simulink model "chap2_2"  (Simulink 3.00)
settings: Solver=ode4  StartTime=0  StopTime=2  FixedStep=0.001  RelTol=1e-3
settings Model: SaveTime=off  SaveOutput=off  LastModifiedBy=liu

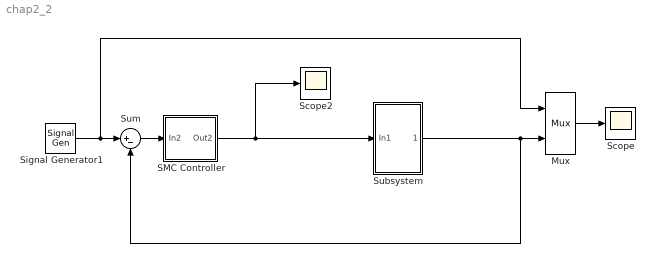
== system chap2_2 ==
  Mux : Mux  Inputs=2
      settings: DisplayOption=none
  SMC Controller : Subsystem
  Scope : Scope
      settings: TimeRange=1  YMin=-0.55  YMax=0.55  SaveName=datas  MaxRows=500000
  Scope2 : Scope
      settings: TimeRange=auto  YMin=-5  YMax=5  SaveToWorkspace=off  SaveName=ScopeData  MaxRows=50000
  Signal Generator1 : SignalGenerator  WaveForm=sine  Amplitude=0.5  Frequency=3  Units=Hertz
  Subsystem : Subsystem
  Sum : Sum  Inputs=|+-  SaturateOnIntegerOverflow=on
  wires:
  Mux/1 -> Scope/1
  SMC Controller/1(Out2) -> Scope2/1, Subsystem/1(In1)
  Signal Generator1/1 -> Sum/1, Mux/1
  Sum/1 -> SMC Controller/1(In2)
  Subsystem/1(Out1) -> Mux/2, Sum/2

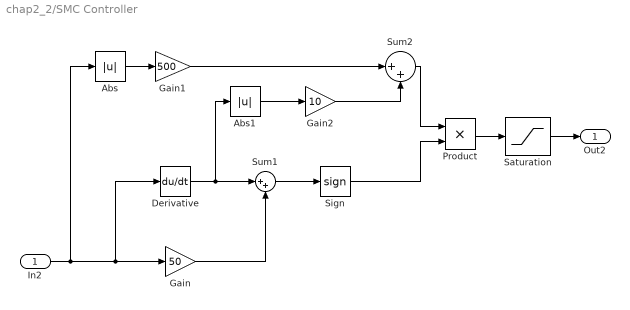
== system chap2_2/SMC Controller ==
  In2 : Inport  Port=1  PortWidth=-1  SampleTime=-1  DataType=auto
      settings: SignalType=auto
  Abs : Abs
  Abs1 : Abs
  Derivative : Derivative
  Gain : Gain  Gain=50  SaturateOnIntegerOverflow=on
  Gain1 : Gain  Gain=500  SaturateOnIntegerOverflow=on
  Gain2 : Gain  Gain=10  SaturateOnIntegerOverflow=on
  Product : Product  Inputs=2  SaturateOnIntegerOverflow=on
  Saturation : Saturate  UpperLimit=110  LowerLimit=-110
  Sign : Signum
  Sum1 : Sum  Inputs=|++  SaturateOnIntegerOverflow=on
  Sum2 : Sum  Inputs=|++  SaturateOnIntegerOverflow=on
  Out2 : Outport  Port=1
  wires:
  Saturation/1 -> Out2/1
  Gain/1 -> Sum1/2
  Sum1/1 -> Sign/1
  Derivative/1 -> Abs1/1, Sum1/1
  Abs1/1 -> Gain2/1
  Gain2/1 -> Sum2/2
  Abs/1 -> Gain1/1
  Gain1/1 -> Sum2/1
  Product/1 -> Saturation/1
  Sum2/1 -> Product/1
  Sign/1 -> Product/2
  In2/1 -> Abs/1, Gain/1, Derivative/1

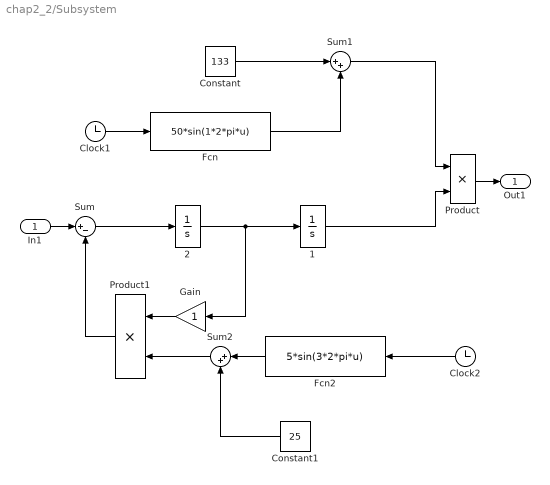
== system chap2_2/Subsystem ==
  In1 : Inport  Port=1  PortWidth=-1  SampleTime=-1  DataType=auto
      settings: SignalType=auto
  " 1" : Integrator  ExternalReset=none  InitialConditionSource=internal  InitialCondition=0  LimitOutput=off  UpperSaturationLimit=inf  LowerSaturationLimit=-inf  ShowSaturationPort=off  ShowStatePort=off  AbsoluteTolerance=auto
  " 2" : Integrator  ExternalReset=none  InitialConditionSource=internal  InitialCondition=0  LimitOutput=off  UpperSaturationLimit=inf  LowerSaturationLimit=-inf  ShowSaturationPort=off  ShowStatePort=off  AbsoluteTolerance=auto
  Clock1 : Clock
  Clock2 : Clock
  Constant : Constant  Value=133
  Constant1 : Constant  Orientation=left  Value=25
  "Fcn " : Fcn  Expr=50*sin(1*2*pi*u)
  Fcn2 : Fcn  Orientation=left  Expr=5*sin(3*2*pi*u)
  Gain : Gain  Orientation=left  Gain=1  SaturateOnIntegerOverflow=on
  Product : Product  Inputs=2  SaturateOnIntegerOverflow=on
  Product1 : Product  Orientation=left  Inputs=2  SaturateOnIntegerOverflow=on
  Sum : Sum  Inputs=|+-  SaturateOnIntegerOverflow=on
  Sum1 : Sum  Inputs=|++  SaturateOnIntegerOverflow=on
  Sum2 : Sum  Orientation=left  Inputs=|++  SaturateOnIntegerOverflow=on
  Out1 : Outport  Port=1
  wires:
  Sum/1 -> " 2"/1
  Clock1/1 -> "Fcn "/1
  " 1"/1 -> Product/2
  " 2"/1 -> " 1"/1, Gain/1
  Clock2/1 -> Fcn2/1
  Gain/1 -> Product1/1
  Product1/1 -> Sum/2
  Product/1 -> Out1/1
  In1/1 -> Sum/1
  "Fcn "/1 -> Sum1/2
  Constant/1 -> Sum1/1
  Sum1/1 -> Product/1
  Fcn2/1 -> Sum2/1
  Sum2/1 -> Product1/2
  Constant1/1 -> Sum2/2
